simulink model "MPC_path_following"  (R2019a)
settings: Solver=VariableStepAuto  StartTime=0.0  StopTime=25  RelTol=1e-3
values from neighbouring files (symbols this model uses):
  A = [A1 zeros(2) ... (first row only)    [MPC_lane_following.m]
  B = [B1 zeros(2,1) ... (first row only)    [MPC_lane_following.m]
  C = [C1 zeros(1,2) ... (first row only)    [MPC_lane_following.m]
  D = [D1 0 ... (first row only)    [MPC_lane_following.m]
undefined symbols (not defined in the file or in its folder): md, Ts
libraries: mpcadaslib x1
settings Model: Creator=VENKAT B  LastModifiedBy=VENKAT B

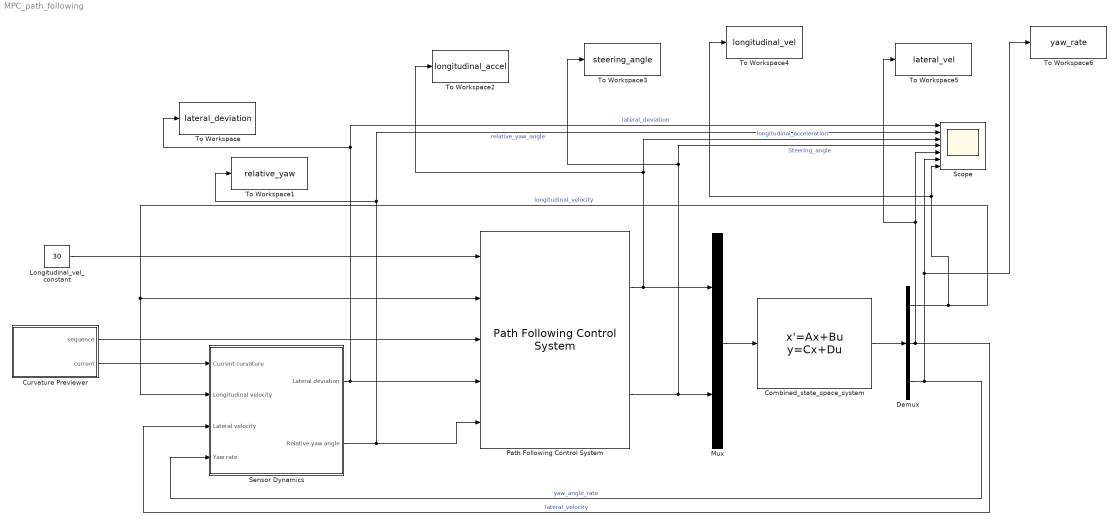
== system MPC_path_following ==
  Combined_state_space_system : StateSpace  A=A  B=B  C=C  D=D  InitialCondition=[0 0.1 0 0]
  Curvature Previewer : Subsystem  mask{signal=md, ts=Ts, steps=10}
      mask prompts: signal "Signal name"; ts "Sampling time"; steps "Number of previewing steps"
      mask init:
      | ts = evalin('base',get_param(gcbh,'ts'));
      | signal = evalin('base',get_param(gcbh,'signal'));
      | steps = evalin('base',get_param(gcbh,'steps'));
      | data = mpc_previewer_maskinit(signal,ts);
      mask Display:
      | fprintf('Future\nsample\nextractor');
      | port_label('output', 1, 'seq')
      | port_label('output', 2, '@t')
  Demux : Demux  Outputs=3
  Longitudinal_vel_constant : Constant  Value=30
  Mux : Mux  Inputs=2
  Path Following Control System : mpcadaslib/Path Following Control System  VariantControl=Variant2  ModelType=Use vehicle parameters  VehicleMass=1575  VehicleYawInertia=2875  LengthToFront=1.2  LengthToRear=1.6  FrontTireStiffness=19000  RearTireStiffness=33000  AccelTimeConstant=0.5  EgoModelMatrixA=[-2,zeros(1,3);1,zeros(1,3);zeros(1,2),-4.4021,-12.4603;zeros(1,2),1.3913,-5.1868]  EgoModelMatrixB=[2,zeros(1,3);zeros(1,2),24.1270,15.8609]'  EgoModelMatrixC=[zeros(3,1),eye(3)]  InitialLongVel=15  TransportLag=0  spaceCtrl=off  DefaultSpacing=10  MinSteering=-0.5  umin_ext=off  MaxSteering=0.5  umax_ext=off  MinAcceleration=-3  amin_ext=off  MaxAcceleration=3  amax_ext=off  Ts=0.1  PredictionHorizon=10  ControlHorizon=3  LongWeight=1  LateralWeight=1  AccelRateWeight=0.1  SteerRateWeight=0.1  suboptimal=off  maxiter=10  datatypeopt=double  optmode=off  trackmode=off
      settings: SourceProductName=MATLAB Runtime - Model Predictive Control Toolbox Addin  SourceProductBaseCode=Missing
  Scope : Scope  NumInputPorts=7
  Sensor Dynamics : Subsystem
  To Workspace : ToWorkspace  VariableName=lateral_deviation  SaveFormat=Timeseries  SampleTime=-1
  To Workspace1 : ToWorkspace  VariableName=relative_yaw  SaveFormat=Timeseries  SampleTime=-1
  To Workspace2 : ToWorkspace  VariableName=longitudinal_accel  SaveFormat=Timeseries  SampleTime=-1
  To Workspace3 : ToWorkspace  VariableName=steering_angle  SaveFormat=Timeseries  SampleTime=-1
  To Workspace4 : ToWorkspace  VariableName=longitudinal_vel  SaveFormat=Timeseries  SampleTime=-1
  To Workspace5 : ToWorkspace  VariableName=lateral_vel  SaveFormat=Timeseries  SampleTime=-1
  To Workspace6 : ToWorkspace  VariableName=yaw_rate  SaveFormat=Timeseries  SampleTime=-1
  wires:
  Combined_state_space_system/1 -> Demux/1
  Path Following Control System/1 -> To Workspace2/1, Scope/3, Mux/1  "longitudinal_acceleration"
  Path Following Control System/2 -> To Workspace3/1, Scope/4, Mux/2  "Steering_angle"
  Mux/1 -> Combined_state_space_system/1
  Demux/1 -> To Workspace4/1, Scope/7, Path Following Control System/2, Sensor Dynamics/2(Longitudinal velocity)  "longitudinal_velocity"
  Longitudinal_vel_constant/1 -> Path Following Control System/1
  Sensor Dynamics/1(Lateral deviation) -> To Workspace/1, Scope/1, Path Following Control System/4  "lateral_deviation"
  Sensor Dynamics/2(Relative yaw angle) -> To Workspace1/1, Scope/2, Path Following Control System/5  "relative_yaw_angle"
  Curvature Previewer/2(current) -> Sensor Dynamics/1(Current curvature)
  Curvature Previewer/1(sequence) -> Path Following Control System/3
  Demux/2 -> Sensor Dynamics/3(Lateral velocity), To Workspace5/1, Scope/5  "lateral_velocity"
  Demux/3 -> Sensor Dynamics/4(Yaw rate), To Workspace6/1, Scope/6  "yaw_angle_rate"

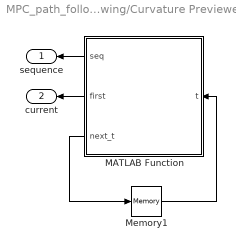
== system MPC_path_following/Curvature Previewer ==
  MATLAB Function : MATLAB Function  TreatAsAtomicUnit=on
  Memory1 : Memory  InheritSampleTime=on  LinearizeAsDelay=on
  sequence : Outport
  current : Outport  Port=2
  wires:
  MATLAB Function/1(seq) -> sequence/1
  MATLAB Function/2(first) -> current/1
  Memory1/1 -> MATLAB Function/1(t)
  MATLAB Function/3(next_t) -> Memory1/1

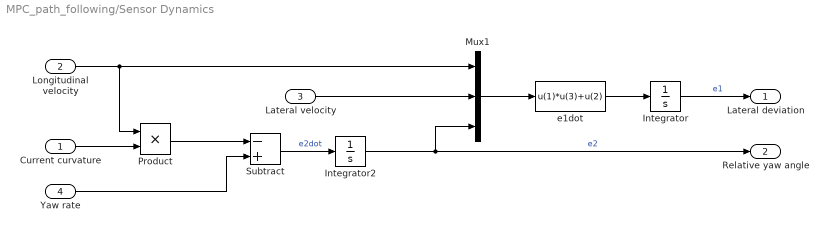
== system MPC_path_following/Sensor Dynamics ==
  Current curvature : Inport
  Longitudinal velocity : Inport  Port=2
  Lateral velocity : Inport  Port=3
  Yaw rate : Inport  Port=4
  Integrator : Integrator
  Integrator2 : Integrator
  Mux1 : Mux  Inputs=[1 1 1]
  Product : Product
  Subtract : Sum  Inputs=-+
  e1dot : Fcn  Expr=u(1)*u(3)+u(2)
  Lateral deviation : Outport
  Relative yaw angle : Outport  Port=2
  wires:
  Current curvature/1 -> Product/2
  Integrator2/1 -> Mux1/3, Relative yaw angle/1  "e2"
  Mux1/1 -> e1dot/1
  e1dot/1 -> Integrator/1
  Longitudinal velocity/1 -> Product/1, Mux1/1
  Lateral velocity/1 -> Mux1/2
  Integrator/1 -> Lateral deviation/1  "e1"
  Product/1 -> Subtract/1
  Yaw rate/1 -> Subtract/2
  Subtract/1 -> Integrator2/1  "e2dot"

== matlab function MPC_path_following/Curvature Previewer/MATLAB Function ==
  settings: updateMethod=DISCRETE  sampleTime=ts
  data: data parameter; seq output; steps parameter; t input; first output; next_t output
function [seq,first,next_t] = fcn(data,steps,t)
%#codegen
[seq,first,next_t] = mpcblock_preview('md',data,steps,t);
